simulink model "dynamicproject"  (R2018b)
settings: Solver=ode45  StartTime=0.0  StopTime=2  RelTol=1e-3
settings Model: Creator=alireza  LastModifiedBy=alireza

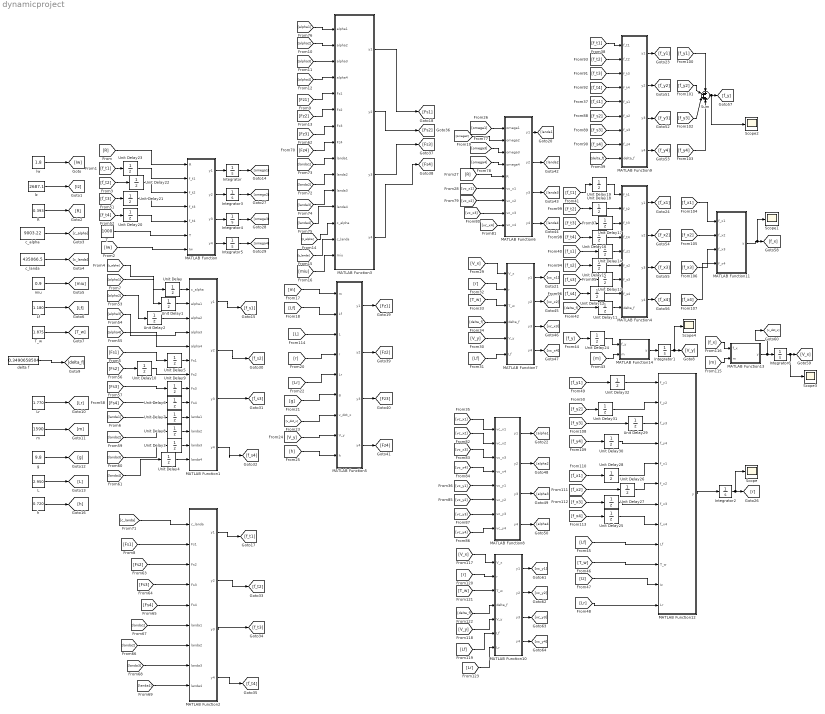
== system dynamicproject ==
  Integrator{,1..6} (7 alike) : Integrator
  L : Constant  Value=2.950
  Lf : Constant  Value=1.180
  Lr : Constant  Value=1.770
  MATLAB Function : MATLAB Function  TreatAsAtomicUnit=on
  MATLAB Function1 : MATLAB Function  TreatAsAtomicUnit=on
  MATLAB Function10 : MATLAB Function  TreatAsAtomicUnit=on
  MATLAB Function11 : MATLAB Function  TreatAsAtomicUnit=on
  MATLAB Function12 : MATLAB Function  TreatAsAtomicUnit=on
  MATLAB Function13 : MATLAB Function  TreatAsAtomicUnit=on
  MATLAB Function14 : MATLAB Function  TreatAsAtomicUnit=on
  MATLAB Function2 : MATLAB Function  TreatAsAtomicUnit=on
  MATLAB Function3 : MATLAB Function  TreatAsAtomicUnit=on
  MATLAB Function4 : MATLAB Function  TreatAsAtomicUnit=on
  MATLAB Function5 : MATLAB Function  TreatAsAtomicUnit=on
  MATLAB Function6 : MATLAB Function  TreatAsAtomicUnit=on
  MATLAB Function7 : MATLAB Function  TreatAsAtomicUnit=on
  MATLAB Function8 : MATLAB Function  TreatAsAtomicUnit=on
  MATLAB Function9 : MATLAB Function  TreatAsAtomicUnit=on
  R : Constant  Value=0.393
  Scope{,1..4} (5 alike) : Scope
  Sum : Sum  Inputs=++++
  T : Constant  Value=1000
  T_w : Constant  Value=1.875
  Unit Delay{,1..32} (33 alike) : UnitDelay  SampleTime=-1
  c_alpha : Constant  Value=9003.22
  c_landa : Constant  Value=435066.5
  delta f : Constant  Value=0.3490658504
  g : Constant  Value=9.8
  h : Constant  Value=0.720
  lw : Constant  Value=1.8
  lz : Constant  Value=2687.1
  m : Constant  Value=1590
  miu : Constant  Value=0.9
  wires:
  lw/1 -> [Iw]
  lz/1 -> [Iz]
  R/1 -> [R]
  c_alpha/1 -> [c_alpha]
  c_landa/1 -> [c_landa]
  miu/1 -> [miu]
  Lf/1 -> [Lf]
  T_w/1 -> [T_w]
  delta f/1 -> [delta_f]
  Lr/1 -> [Lr]
  m/1 -> [m]
  g/1 -> [g]
  L/1 -> [L]
  h/1 -> [h]
  [R] -> MATLAB Function/1(R)
  [f_t1] -> Unit Delay23/1
  T/1 -> MATLAB Function/6(T)
  MATLAB Function/1(y1) -> Integrator/1
  Integrator/1 -> [omega1]
  [c_alpha] -> Unit Delay/1
  [alpha1] -> Unit Delay1/1
  MATLAB Function1/1(y1) -> [f_s1]
  [Lf] -> MATLAB Function5/2(Lf)
  MATLAB Function5/1(y1) -> [Fz1]
  [L] -> MATLAB Function5/3(L)
  [m] -> MATLAB Function5/1(m)
  MATLAB Function6/1(y1) -> [landa1]
  [V_x] -> MATLAB Function7/1(V_x)
  MATLAB Function7/1(y1) -> [vc_x1]
  [vc_x1] -> MATLAB Function8/1(vc_x1)
  MATLAB Function8/1(y1) -> [alpha1]
  MATLAB Function9/1(y1) -> [f_y1]
  Integrator1/1 -> Scope4/1, [V_y]
  MATLAB Function12/1(y) -> Integrator2/1
  Integrator2/1 -> Scope/1, [r]
  [Iw] -> MATLAB Function/7(Iw)
  [f_t2] -> Unit Delay22/1
  [f_t3] -> Unit Delay21/1
  MATLAB Function/2(y2) -> Integrator3/1
  Integrator3/1 -> [omega2]
  MATLAB Function/3(y3) -> Integrator4/1
  Integrator4/1 -> [omega3]
  MATLAB Function/4(y4) -> Integrator5/1
  Integrator5/1 -> [omega4]
  [alpha2] -> Unit Delay2/1
  [alpha3] -> MATLAB Function1/4(alpha3)
  [alpha4] -> MATLAB Function1/5(alpha4)
  [Fs1] -> Unit Delay5/1
  [Fs2] -> Unit Delay10/1
  [Fs3] -> Unit Delay9/1
  [Fs4] -> Unit Delay6/1
  [landa1] -> Unit Delay7/1
  [landa2] -> Unit Delay8/1
  [landa3] -> Unit Delay3/1
  [landa4] -> Unit Delay4/1
  MATLAB Function1/4(y4) -> [f_s4]
  MATLAB Function1/3(y3) -> [f_s3]
  MATLAB Function1/2(y2) -> [f_s2]
  [landa1] -> MATLAB Function2/6(landa1)
  MATLAB Function2/2(y2) -> [f_t2]
  [Fs3] -> MATLAB Function2/4(Fs3)
  [Fs4] -> MATLAB Function2/5(Fs4)
  MATLAB Function2/4(y4) -> [f_t4]
  [Fs1] -> MATLAB Function2/2(Fs1)
  [Fs2] -> MATLAB Function2/3(Fs2)
  [landa4] -> MATLAB Function2/9(landa4)
  MATLAB Function2/1(y1) -> [f_t1]
  MATLAB Function2/3(y3) -> [f_t3]
  [landa2] -> MATLAB Function2/7(landa2)
  [c_landa] -> MATLAB Function2/1(c_landa)
  [landa3] -> MATLAB Function2/8(landa3)
  [miu] -> MATLAB Function3/15(miu)
  [c_landa] -> MATLAB Function3/14(c_landa)
  [c_alpha] -> MATLAB Function3/13(c_alpha)
  [alpha1] -> MATLAB Function3/1(alpha1)
  [alpha2] -> MATLAB Function3/2(alpha2)
  [alpha3] -> MATLAB Function3/3(alpha3)
  [alpha4] -> MATLAB Function3/4(alpha4)
  [Fz1] -> MATLAB Function3/5(Fz1)
  [Fz2] -> MATLAB Function3/6(Fz2)
  [Fz3] -> MATLAB Function3/7(Fz3)
  [Fz4] -> MATLAB Function3/8(Fz4)
  [landa1] -> MATLAB Function3/9(landa1)
  [landa2] -> MATLAB Function3/10(landa2)
  [landa3] -> MATLAB Function3/11(landa3)
  [landa4] -> MATLAB Function3/12(landa4)
  MATLAB Function3/1(y1) -> [Fs1]
  MATLAB Function3/2(y2) -> [Fs2]
  MATLAB Function3/3(y3) -> [Fs3]
  MATLAB Function3/4(y4) -> [Fs4]
  [r] -> MATLAB Function5/4(r)
  [Lr] -> MATLAB Function5/5(Lr)
  [g] -> MATLAB Function5/6(g)
  [v_dot_x] -> MATLAB Function5/7(v_dot_x)
  [V_y] -> MATLAB Function5/8(V_y)
  [h] -> MATLAB Function5/9(h)
  MATLAB Function5/2(y2) -> [Fz2]
  MATLAB Function5/3(y3) -> [Fz3]
  MATLAB Function5/4(y4) -> [Fz4]
  [omega1] -> MATLAB Function6/1(omega1)
  [omega2] -> MATLAB Function6/2(omega2)
  [omega3] -> MATLAB Function6/3(omega3)
  [omega4] -> MATLAB Function6/4(omega4)
  [R] -> MATLAB Function6/5(R)
  [vc_x1] -> MATLAB Function6/6(vc_x1)
  [vc_x4] -> MATLAB Function6/9(vc_x4)
  [vc_x2] -> MATLAB Function6/7(vc_x2)
  [vc_x3] -> MATLAB Function6/8(vc_x3)
  MATLAB Function6/2(y2) -> [landa2]
  MATLAB Function6/3(y3) -> [landa3]
  MATLAB Function6/4(y4) -> [landa4]
  MATLAB Function7/4(y4) -> [vc_x4]
  MATLAB Function7/3(y3) -> [vc_x3]
  MATLAB Function7/2(y2) -> [vc_x2]
  [T_w] -> MATLAB Function7/3(T_w)
  [delta_f] -> MATLAB Function7/4(delta_f)
  [r] -> MATLAB Function7/2(r)
  [V_y] -> MATLAB Function7/5(V_y)
  [Lf] -> MATLAB Function7/6(Lf)
  [vc_x2] -> MATLAB Function8/2(vc_x2)
  [vc_x3] -> MATLAB Function8/3(vc_x3)
  [vc_x4] -> MATLAB Function8/4(vc_x4)
  [vc_y1] -> MATLAB Function8/5(vc_y1)
  [vc_y2] -> MATLAB Function8/6(vc_y2)
  [vc_y3] -> MATLAB Function8/7(vc_y3)
  [vc_y4] -> MATLAB Function8/8(vc_y4)
  MATLAB Function8/2(y2) -> [alpha2]
  MATLAB Function8/3(y3) -> [alpha3]
  MATLAB Function8/4(y4) -> [alpha4]
  [delta_f] -> MATLAB Function9/9(delta_f)
  [f_s1] -> MATLAB Function9/5(f_s1)
  [f_s2] -> MATLAB Function9/6(f_s2)
  [f_s3] -> MATLAB Function9/7(f_s3)
  [f_s4] -> MATLAB Function9/8(f_s4)
  [f_t3] -> MATLAB Function9/3(f_t3)
  [f_t4] -> MATLAB Function9/4(f_t4)
  [f_t2] -> MATLAB Function9/2(f_t2)
  [f_t1] -> MATLAB Function9/1(f_t1)
  MATLAB Function9/2(y2) -> [f_y2]
  MATLAB Function9/3(y3) -> [f_y3]
  MATLAB Function9/4(y4) -> [f_y4]
  [delta_f] -> Unit Delay11/1
  [f_s1] -> Unit Delay14/1
  [f_s2] -> Unit Delay15/1
  [f_t3] -> Unit Delay17/1
  [f_s3] -> Unit Delay13/1
  [f_t4] -> Unit Delay16/1
  MATLAB Function4/3(y3) -> [f_x3]
  MATLAB Function4/2(y2) -> [f_x2]
  [f_t2] -> Unit Delay18/1
  MATLAB Function4/1(y1) -> [f_x1]
  [f_s4] -> Unit Delay12/1
  MATLAB Function4/4(y4) -> [f_x4]
  [f_y4] -> Sum/4
  [f_y3] -> Sum/3
  [f_y2] -> Sum/2
  [f_y1] -> Sum/1
  Sum/1 -> Scope2/1, [f_y]
  [Lr] -> MATLAB Function12/12(Lr)
  [Iz] -> MATLAB Function12/11(Iz)
  [T_w] -> MATLAB Function12/10(T_w)
  [Lf] -> MATLAB Function12/9(Lf)
  [f_x1] -> Unit Delay28/1
  [f_x2] -> Unit Delay26/1
  [f_x3] -> Unit Delay27/1
  [f_x4] -> Unit Delay25/1
  [f_y1] -> Unit Delay32/1
  [f_y2] -> Unit Delay31/1
  [f_y3] -> Unit Delay29/1
  [f_y4] -> Unit Delay30/1
  Integrator6/1 -> Scope3/1, [V_x]
  MATLAB Function10/4(y4) -> [vc_y4]
  [r] -> MATLAB Function10/2(r)
  MATLAB Function10/2(y2) -> [vc_y2]
  MATLAB Function10/3(y3) -> [vc_y3]
  [T_w] -> MATLAB Function10/3(T_w)
  MATLAB Function10/1(y1) -> [vc_y1]
  [V_y] -> MATLAB Function10/5(V_y)
  [V_x] -> MATLAB Function10/1(V_x)
  [Lf] -> MATLAB Function10/6(Lf)
  [delta_f] -> MATLAB Function10/4(delta_f)
  [f_t4] -> Unit Delay20/1
  [Lr] -> MATLAB Function10/7(Lr)
  [f_x1] -> MATLAB Function11/1(f_x1)
  [f_x2] -> MATLAB Function11/2(f_x2)
  [f_x3] -> MATLAB Function11/3(f_x3)
  [f_x4] -> MATLAB Function11/4(f_x4)
  MATLAB Function11/1(y) -> Scope1/1, [f_x]
  [f_x] -> MATLAB Function13/1(f_x)
  [m] -> MATLAB Function13/2(m)
  MATLAB Function13/1(y) -> [v_dot_x], Integrator6/1
  MATLAB Function14/1(y) -> Integrator1/1
  [m] -> MATLAB Function14/2(m)
  Unit Delay/1 -> MATLAB Function1/1(c_alpha)
  Unit Delay1/1 -> MATLAB Function1/2(alpha1)
  Unit Delay5/1 -> MATLAB Function1/6(Fs1)
  Unit Delay4/1 -> MATLAB Function1/13(landa4)
  Unit Delay3/1 -> MATLAB Function1/12(landa3)
  Unit Delay2/1 -> MATLAB Function1/3(alpha2)
  Unit Delay8/1 -> MATLAB Function1/11(landa2)
  Unit Delay7/1 -> MATLAB Function1/10(landa1)
  Unit Delay6/1 -> MATLAB Function1/9(Fs4)
  Unit Delay9/1 -> MATLAB Function1/8(Fs3)
  Unit Delay10/1 -> MATLAB Function1/7(Fs2)
  Unit Delay11/1 -> MATLAB Function4/9(delta_f)
  Unit Delay12/1 -> MATLAB Function4/8(f_s4)
  Unit Delay13/1 -> MATLAB Function4/7(f_s3)
  Unit Delay15/1 -> MATLAB Function4/6(f_s2)
  Unit Delay14/1 -> MATLAB Function4/5(f_s1)
  Unit Delay16/1 -> MATLAB Function4/4(f_t4)
  Unit Delay17/1 -> MATLAB Function4/3(f_t3)
  Unit Delay18/1 -> MATLAB Function4/2(f_t2)
  [f_t1] -> Unit Delay19/1
  Unit Delay19/1 -> MATLAB Function4/1(f_t1)
  Unit Delay20/1 -> MATLAB Function/5(f_t4)
  Unit Delay21/1 -> MATLAB Function/4(f_t3)
  Unit Delay22/1 -> MATLAB Function/3(f_t2)
  Unit Delay23/1 -> MATLAB Function/2(f_t1)
  [f_y] -> Unit Delay24/1
  Unit Delay24/1 -> MATLAB Function14/1(f_y)
  Unit Delay25/1 -> MATLAB Function12/8(f_x4)
  Unit Delay27/1 -> MATLAB Function12/7(f_x3)
  Unit Delay26/1 -> MATLAB Function12/6(f_x2)
  Unit Delay28/1 -> MATLAB Function12/5(f_x1)
  Unit Delay30/1 -> MATLAB Function12/4(f_y4)
  Unit Delay29/1 -> MATLAB Function12/3(f_y3)
  Unit Delay31/1 -> MATLAB Function12/2(f_y2)
  Unit Delay32/1 -> MATLAB Function12/1(f_y1)

== matlab function dynamicproject/MATLAB Function1 ==
  data: c_alpha input; y1 output; alpha1 input; alpha2 input; alpha3 input; alpha4 input; Fs1 input; Fs2 input; Fs3 input; Fs4 input; landa1 input; landa2 input; landa3 input; landa4 input; y2 output; y3 output; y4 output
function [y1,y2,y3,y4] = f_s(c_alpha,alpha1,alpha2,alpha3,alpha4,Fs1,Fs2,Fs3,Fs4,landa1,landa2,landa3,landa4)
 landa=[landa1,landa2,landa3,landa4];
  alpha=[alpha1 alpha2 alpha3 alpha4];
  Fs=[Fs1,Fs2,Fs3,Fs4];
  f_s=zeros(1,4);
for i=1:4
   
    f_s(i)=((c_alpha*alpha(i))/(1+landa(i)))*Fs(i);
end

y1 = f_s(1);
y2= f_s(2);
y3= f_s(3);
y4= f_s(4);

== matlab function dynamicproject/MATLAB Function ==
  data: R input; y1 output; f_t1 input; f_t2 input; f_t3 input; f_t4 input; T input; y2 output; y3 output; y4 output; Iw input
function [y1,y2,y3,y4]= omega(R,f_t1,f_t2,f_t3,f_t4,T,Iw)
omega_dot=zeros(1,4);
f_t=[f_t1,f_t2,f_t3,f_t4];
for i=1:4
omega_dot(i)=(T-f_t(i)*R)/Iw;
end
y1 = omega_dot(1);
y2 = omega_dot(2);
y3 = omega_dot(3);
y4 = omega_dot(4);

== matlab function dynamicproject/MATLAB Function2 ==
  data: c_landa input; y1 output; Fs1 input; Fs2 input; Fs3 input; Fs4 input; landa1 input; landa2 input; landa3 input; landa4 input; y2 output; y3 output; y4 output
function [y1,y2,y3,y4] = f_t(c_landa,Fs1,Fs2,Fs3,Fs4,landa1,landa2,landa3,landa4)
 landa=[landa1,landa2,landa3,landa4];
  Fs=[Fs1,Fs2,Fs3,Fs4];
   f_t=zeros(1,4);
for i=1:4
   
    f_t(i)=((c_landa*landa(i))/(1+landa(i)))*Fs(i);
end

y1 = f_t(1);
y2= f_t(2);
y3= f_t(3);
y4= f_t(4);

== matlab function dynamicproject/MATLAB Function3 ==
  data: alpha1 input; y1 output; alpha2 input; alpha3 input; alpha4 input; Fz1 input; Fz2 input; Fz3 input; Fz4 input; landa1 input; landa2 input; landa3 input; landa4 input; c_alpha input; c_landa input; miu input; y2 output; y3 output; y4 output
function [y1,y2,y3,y4] = Fs(alpha1,alpha2,alpha3,alpha4,Fz1,Fz2,Fz3,Fz4,landa1,landa2,landa3,landa4,c_alpha,c_landa,miu)
landa=[landa1,landa2,landa3,landa4];
alpha=[alpha1 alpha2 alpha3 alpha4];
 Fz=[Fz1 Fz2 Fz3 Fz4];
  Fs=zeros(1,4);
  s=zeros(1,4);
for i=1:4
   
    s(i)=((miu*Fz(i)*(1+landa(i)))/(2*sqrt((c_landa*landa(i))^2+(c_alpha*tan(alpha(i)))^2)));
if s(i)<1
    Fs(i)=(2-s(i))*s(i);
else
    Fs(i)=1;
end
end
y1=Fs(1);
y2=Fs(2);
y3=Fs(3);
y4=Fs(4);

== matlab function dynamicproject/MATLAB Function4 ==
  data: f_t1 input; y1 output; f_t2 input; f_t3 input; f_t4 input; f_s1 input; f_s2 input; f_s3 input; f_s4 input; delta_f input; y2 output; y3 output; y4 output
function [y1,y2,y3,y4] = f_x(f_t1,f_t2,f_t3,f_t4,f_s1,f_s2,f_s3,f_s4,delta_f)
f_t=[f_t1,f_t2,f_t3,f_t4];
f_s=[f_s1,f_s2,f_s3,f_s4];
f_x=zeros(1,4);
for i=1:4
    f_x(i)=f_t(i)*cos(delta_f)-f_s(i)*sin(delta_f);
end
y1 = f_x(1);
y2 = f_x(2);
y3 = f_x(3);
y4 = f_x(4);

== matlab function dynamicproject/MATLAB Function5 ==
  data: m input; y1 output; Lf input; L input; r input; Lr input; g input; v_dot_x input; V_y input; h input; y2 output; y3 output; y4 output
function [y1,y2,y3,y4]=Fz(m,Lf,L,r,Lr,g,v_dot_x,V_y,h)
Fz=zeros(1,4);
for i=1:2
    Fz(i)=(m*g/2)*(Lr/(2*L)-((v_dot_x-V_y*r)*h/(g*L)));
end
for i=3:4
    Fz(i)=(m*g/2)*(Lf/L+((v_dot_x-V_y*r)*h/(g*L)));
end
y1 =Fz(1);
y2 =Fz(2) ;
y3 =Fz(3) ;
y4 =Fz(4) ;

== matlab function dynamicproject/MATLAB Function6 ==
  data: omega1 input; y1 output; omega2 input; omega3 input; omega4 input; R input; vc_x1 input; vc_x2 input; vc_x3 input; vc_x4 input; y2 output; y3 output; y4 output
function [y1,y2,y3,y4] = landa(omega1,omega2,omega3,omega4,R,vc_x1,vc_x2,vc_x3,vc_x4)
omega=[omega1,omega2,omega3,omega4];
vc_x=[vc_x1,vc_x2,vc_x3,vc_x4];
landa=zeros(1,4);
for i=1:4
    landa(i)= (omega(i)*R-vc_x(i))/vc_x(i);
end
y1 =landa(1);
y2 =landa(2);
y3 =landa(3);
y4 =landa(4);

== matlab function dynamicproject/MATLAB Function7 ==
  data: V_x input; y1 output; r input; T_w input; delta_f input; V_y input; Lf input; y2 output; y3 output; y4 output
function [y1,y2,y3,y4] = Vc_x(V_x,r,T_w,delta_f,V_y,Lf)

y1 =(V_x-r*T_w/2)*cos(delta_f)+(V_y+r*Lf)*sin(delta_f);
y2 =(V_x+r*T_w/2)*cos(delta_f)+(V_y+r*Lf)*sin(delta_f);
y3=V_x-r*T_w/2;
y4=V_x+r*T_w/2;

== matlab function dynamicproject/MATLAB Function8 ==
  data: vc_x1 input; y1 output; vc_x2 input; vc_x3 input; vc_x4 input; vc_y1 input; vc_y2 input; vc_y3 input; vc_y4 input; y2 output; y3 output; y4 output
function [y1,y2,y3,y4] = alpha(vc_x1,vc_x2,vc_x3,vc_x4,vc_y1,vc_y2,vc_y3,vc_y4)
vc_x=[vc_x1,vc_x2,vc_x3,vc_x4];
vc_y=[vc_y1,vc_y2,vc_y3,vc_y4];
alpha=zeros(1,4);
for i=1:4
    alpha(i)=atan2(vc_y(i),vc_x(i));
end

y1=alpha(1);
y2=alpha(2);
y3=alpha(3);
y4=alpha(4);

== matlab function dynamicproject/MATLAB Function9 ==
  data: f_t1 input; y1 output; f_t2 input; f_t3 input; f_t4 input; f_s1 input; f_s2 input; f_s3 input; f_s4 input; delta_f input; y2 output; y3 output; y4 output
function [y1,y2,y3,y4] = f_y(f_t1,f_t2,f_t3,f_t4,f_s1,f_s2,f_s3,f_s4,delta_f)
f_t=[f_t1,f_t2,f_t3,f_t4];
f_s=[f_s1,f_s2,f_s3,f_s4];
f_y=[0 0 0 0];
for i=1:4
    f_y(i)=f_t(i)*sin(delta_f)+f_s(i)*cos(delta_f);
end
y1 = f_y(1);
y2 = f_y(2);
y3 = f_y(3);
y4 = f_y(4);

== matlab function dynamicproject/MATLAB Function10 ==
  data: V_x input; y1 output; r input; T_w input; delta_f input; V_y input; Lf input; y2 output; y3 output; y4 output; Lr input
function [y1,y2,y3,y4]=vcy(V_x,r,T_w,delta_f,V_y,Lf,Lr)
vcy=zeros(1,4);
y1=0;
y2=0;
y3=0;
y4=0;
vcy(1) =(-V_x+r*T_w/2)*sin(delta_f)+(V_y+r*Lf)*cos(delta_f);
vcy(2) =(-V_x-r*T_w/2)*sin(delta_f)+(V_y+r*Lf)*cos(delta_f);
vcy(3)=V_y+r*Lr;
vcy(4)=V_y+r*Lr;
y1=vcy(1);
y2=vcy(2);
y3=vcy(3);
y4=vcy(4);

== matlab function dynamicproject/MATLAB Function11 ==
  data: f_x1 input; y output; f_x2 input; f_x3 input; f_x4 input
function y = fcn(f_x1,f_x2,f_x3,f_x4)


y =f_x1+f_x2+f_x3+f_x4 ;

== matlab function dynamicproject/MATLAB Function12 ==
  data: f_y1 input; f_y2 input; f_y3 input; y output; f_y4 input; f_x1 input; f_x2 input; f_x3 input; f_x4 input; Lf input; T_w input; Iz input; Lr input
function y =r_dot(f_y1,f_y2,f_y3,f_y4,f_x1,f_x2,f_x3,f_x4,Lf,T_w,Iz,Lr)
r_dot=(Lf*(f_y1+f_y2)-Lr*(f_y3+f_y4)+(f_x1+f_x3-f_x2-f_x4)*T_w/2)/Iz;

y = r_dot;

== matlab function dynamicproject/MATLAB Function13 ==
  data: f_x input; y output; m input
function y = fcn(f_x,m)

y = f_x/m;

== matlab function dynamicproject/MATLAB Function14 ==
  data: f_y input; y output; m input
function y = fcn(f_y,m)

y = f_y/m;
